simulink model "HexrotorDynamicModel_2015a"  (Simulink 8.5)
settings: Solver=ode45  SolverMode=SingleTasking  StartTime=0.0  StopTime=10  FixedStep=0.0001  RelTol=1e-3
values from neighbouring files (symbols this model uses):
  alpha = pi/180 * 13.6    (= 0.237364778271)    [IdealParameter.m]    (also in ParLuk11.m = deg2rad(13.6); Parameter.m = [-alpha_i;alpha_i;-alpha_i;alpha_i;-alpha_i;alpha_i]; ParameterIdeal.m = [-alpha_i;alpha_i;-alpha_i;alpha_i;-alpha_i;alpha_i]; ParameterVIVE.m = [alpha_i;-alpha_i;alpha_i;-alpha_i;alpha_i;-alpha_i])
  b = 1.1e-06    [IdealParameter.m]    (also in ParLuk11.m = 1.14e-07; Parameter.m = 8.944e-07; ParameterIdeal.m; ParameterVIVE.m)
  beta = 0    [IdealParameter.m]    (also in ParLuk11.m; Parameter.m = [beta_i; beta_i; beta_i; beta_i; beta_i; beta_i]; ParameterIdeal.m = [beta_i; beta_i; beta_i; beta_i; beta_i; beta_i]; ParameterVIVE.m = [beta_i; beta_i; beta_i; beta_i; beta_i; beta_i])
  g = 9.81    [IdealParameter.m]    (also in ParLuk11.m; Parameter.m; ParameterIdeal.m; ParameterVIVE.m)
  IB = [Ixx 0 0; 0 Iyy 0; 0 0 Izz]    [IdealParameter.m]    (also in ParLuk11.m; Parameter.m; ParameterIdeal.m; ParameterVIVE.m)
  k = 5.6e-05    [IdealParameter.m]    (also in ParLuk11.m = 2.98e-06; Parameter.m = 4.472e-05; ParameterIdeal.m; ParameterVIVE.m = 5.13e-05)
  k_ad = 4    [ParLuk11.m]
  k_ap = 2    [ParLuk11.m]
  K_d = diag([5,5,5,6,6,6])    [ParLuk11.m]
  K_p1 = 10*eye(3)    [ParLuk11.m]
  k_p2 = 6    [ParLuk11.m]
  K_P_1 = 15*eye(3)    [IdealParameter.m]    (also in ParLuk11.m = 6*eye(3); Parameter.m = 2*eye(3); ParameterIdeal.m; ParameterVIVE.m = 10*eye(3))
  K_P_2 = 50*eye(3)    [IdealParameter.m]    (also in ParLuk11.m = 6*eye(3); Parameter.m = 4*eye(3); ParameterIdeal.m; ParameterVIVE.m = 10*eye(3))
  K_P_3 = 60*eye(3)    [IdealParameter.m]    (also in ParLuk11.m = 6*eye(3); Parameter.m = 6*eye(3); ParameterIdeal.m; ParameterVIVE.m = 10*eye(3))
  K_P_D = 30*eye(3)    [IdealParameter.m]    (also in ParLuk11.m = 10*eye(3); Parameter.m = 5*eye(3); ParameterIdeal.m; ParameterVIVE.m = 15*eye(3))
  K_P_I = 100*eye(3)    [IdealParameter.m]    (also in ParLuk11.m = 10*eye(3); Parameter.m = 10*eye(3); ParameterIdeal.m = 80*eye(3); ParameterVIVE.m)
  K_P_P = 100*eye(3)    [IdealParameter.m]    (also in ParLuk11.m = 10*eye(3); Parameter.m = 10*eye(3); ParameterIdeal.m = 130*eye(3); ParameterVIVE.m)
  k_pd = 8    [ParLuk11.m]
  k_pp = 4    [ParLuk11.m]
  K_R_1 = 40*eye(3)    [IdealParameter.m]    (also in ParLuk11.m = 3*eye(3); Parameter.m = 2*eye(3); ParameterIdeal.m; ParameterVIVE.m = 10*eye(3))
  K_R_2 = 100*eye(3)    [IdealParameter.m]    (also in ParLuk11.m = 3*eye(3); Parameter.m = 4*eye(3); ParameterIdeal.m; ParameterVIVE.m = 10*eye(3))
  K_R_3 = 50*eye(4)    [IdealParameter.m]    (also in ParLuk11.m = eye(4); Parameter.m = 6*eye(4); ParameterIdeal.m; ParameterVIVE.m = 10*eye(4))
  K_R_D = 30*eye(3)    [IdealParameter.m]    (also in ParLuk11.m = 10*eye(3); Parameter.m = 5*eye(3); ParameterIdeal.m; ParameterVIVE.m = 15*eye(3))
  K_R_I = 100*eye(3)    [IdealParameter.m]    (also in ParLuk11.m = 10*eye(3); Parameter.m = 10*eye(3); ParameterIdeal.m = 80*eye(3); ParameterVIVE.m)
  K_R_P = 100*eye(3)    [IdealParameter.m]    (also in ParLuk11.m = 20*eye(3); Parameter.m = 10*eye(3); ParameterIdeal.m = 130*eye(3); ParameterVIVE.m)
  k_z = 15    [ParLuk11.m]
  L = 0.4    [IdealParameter.m]    (also in ParLuk11.m = 1; Parameter.m; ParameterIdeal.m; ParameterVIVE.m = 0.6)
  m = 1    [Controllability.m]    (also in IdealParameter.m = 2.5; ParLuk11.m = 0.6; Parameter.m = 4.85; ParameterIdeal.m = 4.85)
libraries: vrlib x8, simulink x3, dspmtrx3 x2
(part 2 of 2)

== matlab function Motion Equations/MATLAB Function1 ==
  data: w input double; Q output double
function Q = omegaSkew(w)
%#codegen

Q = [0 w(3) -w(2) w(1);
    -w(3) 0 w(1) w(2);
    w(2) -w(1) 0 w(3);
    -w(1) -w(2) -w(3) 0];

== matlab function Motion Equations/MATLAB Function2 ==
  data: R input double; RT output double
function RT = transpose(R)
%#codegen

RT = R';

== matlab function Feedback Linearization Control [Raj15]/MATLAB Function1 ==
  data: R_m input double; JR output double; I_B input double
function JR = computeJR(R_m, I_B)
JR = [R_m zeros(3);
     zeros(3) inv(I_B) ];

== matlab function Geometric Control on SE(3) [Ras17]/MATLAB Function ==
  data: W_g input double; W_ff output double; I input double; T_B input double; T_D input double; T_D_dot input double; H_er input double
function W_ff = computeW_ff(W_g, I, T_B, T_D, T_D_dot, H_er)

R_er = H_er(1:3,1:3);
eta_er = H_er(1:3,4);

%H_er_inv = [R_er', -R_er'*eta_er; 0,0,0,1];

Ad_H_er_inv = [R_er', zeros(3);
               vec2skew(-R_er'*eta_er)*R_er', R_er'];

T_er = T_B - Ad_H_er_inv*T_D;

ad_T_er = [vec2skew(T_er(1:3)), zeros(3);
            vec2skew(T_er(4:6)), vec2skew(T_er(1:3))];
        
ad_T_B = [vec2skew(T_B(1:3)), zeros(3);
    vec2skew(T_B(4:6)), vec2skew(T_B(1:3))];
        
W_ff =  - W_g ...
        - ad_T_B' * (I*T_B) ...
        + I * ( Ad_H_er_inv * T_D_dot - ad_T_er * Ad_H_er_inv * T_D);

== matlab function Geometric Control on SE(3) [Ras17]/MATLAB Function1 ==
  data: R_BtoI input double; g input double; W_g output double; m input double
function W_g = computeW_g(R_BtoI, g, m)

W_g = [R_BtoI', zeros(3);
        zeros(3), R_BtoI'] * [0,0,0,0,0,-m*g]';

== matlab function MATLAB Function2 ==
  data: t input double; p_d output double; p_d_dot output double; p_d_dotdot output double; R_d output double; omega_d output double; omega_d_dot output double; T_D output double; T_D_dot output double
function [p_d, p_d_dot, p_d_dotdot, R_d, omega_d, omega_d_dot, T_D, T_D_dot] = createTrajectory(t)

xa = 0;
xe = 5;
te = 5;
x = xa + 10*(xe-xa)*t^3/te^3 - 15*(xe-xa)*t^4/te^4 + 6*(xe-xa)*t^5/te^5;
x_dot = 3*10*(xe-xa)*t^2/te^3 - 4*15*(xe-xa)*t^3/te^4 + 5*6*(xe-xa)*t^4/te^5;
x_dot_dot = 6*10*(xe-xa)*t/te^3 - 12*15*(xe-xa)*t^2/te^4 + 20*6*(xe-xa)*t^3/te^5;
if (t> te)
    x = xe;
    x_dot = 0;
    x_dot_dot = 0;
end
p_d = [x;0;x];
p_d_dot = [x_dot;0;x_dot];
p_d_dotdot = [x_dot_dot;0;x_dot_dot];

ct = cos(2*pi/te*t);
st = sin(2*pi/te*t);
R_d = [ct, -st, 0; 
       st, ct, 0;
       0 0 1];
R_d_dot = [-st, -ct, 0;
            ct, -st, 0;
            0 0 0];
R_d_dotdot = [-ct, st, 0;
               -st, -ct, 0;
               0 0 0];
           
T_d_tilde = [R_d', -R_d'*p_d; 0,0,0,1]*[R_d_dot p_d_dot; 0,0,0,0];

omega_d = skew2vec(T_d_tilde(1:3,1:3));

T_d_tilde_dot = [R_d_dot'*R_d_dot+R_d'*R_d_dotdot, R_d_dot'*p_d_dot+R_d'*p_d_dotdot;
    0,0,0,0];

omega_d_dot = skew2vec(T_d_tilde_dot(1:3,1:3));

T_D = [omega_d; T_d_tilde(1:3,4)];
T_D_dot = [omega_d_dot; T_d_tilde_dot(1:3,4)];

if t>te
    R_d = eye(3);
    omega_d = [0;0;0];
    omega_d_dot = [0;0;0];
    T_D = zeros(6,1);
    T_D_dot = zeros(6,1);
end

%zeros
% 
% p_d = [0;0;0];
% p_d_dot = [0;0;0];
% p_d_dotdot = [0;0;0];
% R_d = eye(3);
% omega_d = [0;0;0];
% omega_d_dot = [0;0;0];
% T_D = zeros(6,1);
% T_D_dot = zeros(6,1);

== matlab function Geometric Control on SE(3) [Ras17]/MATLAB Function2 ==
  data: m input double; IB input double; I output double
function I = computeI(m, IB)

I = [IB, zeros(3); 
    zeros(3), eye(3)*m];

== matlab function Geometric Control on SE(3) [Ras17]/MATLAB Function3 ==
  data: R_BtoI input double; v_I input double; T_B output double; omega_B input double
function T_B = computeTB(R_BtoI, v_I, omega_B)

T_B = [omega_B;
    R_BtoI' * v_I];

== matlab function DC Motor Dynamics /MATLAB Function ==
  data: u input double; y output double
function y = fcn(u)

y = sqrt(abs(u))*sign(u);

== matlab function DC Motor Dynamics /MATLAB Function1 ==
  data: u input double; y output double
function y = fcn(u)

y = u^2*sign(u);

== matlab function DC Motor Dynamics /MATLAB Function2 ==
  data: u input double; y output double
function y = fcn(u)

y = sqrt(abs(u))*sign(u);

== matlab function DC Motor Dynamics /MATLAB Function3 ==
  data: u input double; y output double
function y = fcn(u)

y = u^2*sign(u);

== matlab function Feedback Linearization Control [Raj15]/MATLAB Function3 ==
  data: u input double; y output double
function y = transpose(u)

y = u';

== matlab function Feedback Linearization Control [Raj15]/MATLAB Function5 ==
  data: R_d input double; e_R output double; R_BtoI input double
function e_R = compute_e_R(R_d, R_BtoI)

A = R_d' * R_BtoI - R_BtoI' * R_d;

e_R = 0.5 * [A(3,2); A(1,3); A(2,1)];

== matlab function Geometric Control on SE(3) [Ras17]/MATLAB Function4 ==
  data: R_BtoI input double; H_er output double; R_d input double; p_I input double; p_d input double
function H_er = computeH_er(R_BtoI, R_d, p_I, p_d)

H_er = [R_d'*R_BtoI, R_d'*(p_I-p_d); 0,0,0,1];

== matlab function Geometric Control on SE(3) [Ras17]/MATLAB Function5 ==
  data: H_er input double; K_p1 input double; W_p output double; kp2 input double
function W_p = computeW_p(H_er, K_p1, kp2)

R_er = H_er(1:3,1:3);
eta_er = H_er(1:3,4);

W_p = - [skew2vec(0.5*(K_p1*R_er-(K_p1*R_er)'));
        -kp2*R_er'*eta_er];

== matlab function Geometric Control on SE(3) [Ras17]/MATLAB Function6 ==
  data: T_B input double; T_er output double; H_er input double; T_D input double
function T_er = computeT_er(T_B, H_er, T_D)

R_er = H_er(1:3,1:3);
eta_er = H_er(1:3,4);

Ad_H_er_inv = [R_er', zeros(3);
               vec2skew(-R_er'*eta_er)*R_er', R_er'];
           
T_er = T_B - Ad_H_er_inv * T_D;

== matlab function Geometric Control on SE(3) [Ras17]/MATLAB Function7 ==
  data: T_er input double; W_d output double; K_d input double
function W_d = compute_Wd(T_er,K_d)

W_d = - K_d * T_er;

== matlab function Geometric Control on SE(3) [Ras17]/MATLAB Function8 ==
  data: W input double; FH input double; u output double
function u = mapToRotors(W,FH)

u = inv(FH)*W;

== matlab function Motion Equations [Ras17]/MATLAB Function1 ==
  data: R_BtoI input double; g input double; W_g output double; m input double
function W_g = computeW_g(R_BtoI, g, m)

W_g = [R_BtoI', zeros(3);
        zeros(3), R_BtoI'] * [0,0,0,0,0,-m*g]';

== matlab function Motion Equations [Ras17]/MATLAB Function2 ==
  data: m input double; IB input double; I output double
function I = computeI(m, IB)

I = [IB, zeros(3); 
    zeros(3), eye(3)*m];

== matlab function Motion Equations [Ras17]/MATLAB Function ==
  data: I input double; Iinv output double
function Iinv = computeInverse(I)
Iinv = inv(I);

== matlab function Motion Equations [Ras17]/MATLAB Function3 ==
  data: T_B input double; ad_T_B output double
function ad_T_B = compute_ad_T_B(T_B)
ad_T_B = [vec2skew(T_B(1:3)), zeros(3);
    vec2skew(T_B(4:6)), vec2skew(T_B(1:3))]';

== matlab function Motion Equations [Ras17]/MATLAB Function4 ==
  data: R input double; RT output double
function RT = transpose(R)
%#codegen

RT = R';

== matlab function Motion Equations [Ras17]/MATLAB Function5 ==
  data: T input double; T_tilde output double
function T_tilde = computeT_tilde(T)

T_tilde = [vec2skew(T(1:3)), T(4:6); 0,0,0,0];

== matlab function Motion Equations [Ras17]/MATLAB Function6 ==
  data: H input double; R_BtoI output double; eta_BtoI output double
function [R_BtoI, eta_BtoI] = computeRandeta(H)

R_BtoI = H(1:3,1:3);
eta_BtoI = H(1:3,4);

== matlab function Zero Moment Control [Mic17] unfertig/MATLAB Function ==
  data: F1 input double; d output double; b2 output double; F2 input double; F2K output double
function [d,b2, F2K] = fcn(F1,F2)
    % null space of F2 or H: 
    % w01 = [1 0 0 1 0 0]', w02 = [0 1 0 0 1 0]', w03 = [0 0 1 0 0 1]'
    b2 = [1 1 1 1 1 1]'*1/2.4495;
    d = F1*b2;

    %null space of F1
    K1 = [-1 0 0; 0 -1 0; 0 0 -1; 1 0 0; 0 1 0; 0 0 1];
    
    % K = K1*K1'
    
    K = K1*K1';
    
    %K*F2'*inv(F2*K*F2');
    F2K = K*F2'/(F2*K*F2');

== matlab function Zero Moment Control [Mic17] unfertig/MATLAB Function1 ==
  data: w_d input double; Q output double
function Q = omegaSkew(w_d)
%#codegen

Q = [0 w_d(3) -w_d(2) w_d(1);
    -w_d(3) 0 w_d(1) w_d(2);
    w_d(2) -w_d(1) 0 w_d(3);
    -w_d(1) -w_d(2) -w_d(3) 0];

== matlab function Zero Moment Control [Mic17] unfertig/MATLAB Function2 ==
  data: q input double; R output double
function R = Quat2R(q)
% compute R from quaternion input

R = [q(1)^2 - q(2)^2 - q(3)^2 + q(4)^2,  2*(q(1)*q(2) - q(3)*q(4)),          2*(q(1)*q(3) + q(2)*q(4));
     2*(q(1)*q(2) + q(3)*q(4)),         -q(1)^2 + q(2)^2 - q(3)^2 + q(4)^2,  2*(q(2)*q(3) - q(1)*q(4));
     2*(q(1)*q(3) - q(2)*q(4)),          2*(q(2)*q(3) + q(1)*q(4)),         -q(1)^2 - q(2)^2 + q(3)^2 + q(4)^2];

== matlab function Zero Moment Control [Mic17] unfertig/MATLAB Function3 ==
  data: R input double; RT output double
function RT = transpose(R)
%#codegen

RT = R';

== matlab function Zero Moment Control [Mic17] unfertig/MATLAB Function4 ==
  data: f_p input double; w_d output double; Rqd input double; u_z input double
function w_d = compute_w_d(f_p, Rqd, u_z)

if f_p == 0
    f_p = 0.0001;
end
w_d = 1/f_p * vec2skew(Rqd) * u_z;

== matlab function Zero Moment Control [Mic17] unfertig/MATLAB Function5 ==
  data: k_pd input double; u_z output double; k_pp input double; k_z input double; m input double; e_p input double; e_v input double; z input double; d input double
function u_z = compute_u_z(k_pd, k_pp, k_z, m, e_p, e_v, z, d)

u_z = (k_pd*k_pp/m*e_p + (k_pd^2/m - k_pp)*e_v + (k_pd/m - k_z)*z)/norm(d, 2)^2;

== matlab function Zero Moment Control [Mic17] unfertig/MATLAB Function6 ==
  data: q input double; delta_q output double; q_d input double
function delta_q = compute_deltaq(q, q_d)

eps_d = q_d(1:3);
n_d = q_d(4);
eps_q = q(1:3);
n_q = q(4);

delta_n = n_d*n_q + eps_d'*eps_q;
delta_eps = -n_q*eps_d + n_d*eps_q - vec2skew(eps_d)*eps_q;

delta_q = [delta_eps; delta_n];

== matlab function Zero Moment Control [Mic17] unfertig/MATLAB Function7 ==
  data: f_p input double; w_dd output double; R_qd input double; d input double; k_pd input double; k_pp input double; m input double; R_q input double; e_p input double; e_v input double; kz input double; z input double
function w_dd = compute_wdd(f_p,R_qd,d, k_pd, k_pp, m, R_q, e_p, e_v, kz,z)

x = (k_pd^2/m^2 - k_pp/m)*(R_q*d*f_p-k_pp*e_p) + ...
    (2*k_pp*k_pd/m - k_pd^3/m^2)*e_v + (k_pd^2/m^2 - k_pp/m - k_pd*kz/m + kz^2)*z;

w_dd = 1/f_p *1/(norm(d)^2) * vec2skew(R_qd*d) * x;

== matlab function Zero Moment Control [Mic17] unfertig/MATLAB Function8 ==
  data: k_ap input double; tau_r output double; k_ad input double; q_delta input double; Rq input double; w_d input double; w input double; J input double; w_dd input double
function tau_r = compute_tau_r(k_ap, k_ad, q_delta, Rq, w_d, w, J, w_dd)

delta_eps = q_delta(1:3);

tau_r = -k_ap*delta_eps - k_ad * (w - Rq'*w_d) + cross(w, J*w) ...
    - J*vec2skew(w)*Rq'*w_d + J*Rq'*w_dd;

== matlab function Integral Backstepping/MATLAB Function1 ==
  data: R input double; q output double
function q   = DCM2Quat(R)

%%%%%%%%%%%%%%%%%%%%%%%%%%%%%%%%%%%%%%%%%%%%%%%%%%%%%%%%%%%%%%%%%%%%%%%%%%%
%
% M-file: Tool_DCM2Quat
%         -> impelmeted as M-Function
% Author: Marcel Tkocz
% Version: 27.01.2008
%
% Description:
%   This Function converts roll-pitch-yaw angels into their quaternion
%   equivalents.
%
% Inputs:
%   Orientation ... orientation in roll-pitch-yaw angels
%
% Outputs:
%   q           ... orientation in quaternions
%   
%%%%%%%%%%%%%%%%%%%%%%%%%%%%%%%%%%%%%%%%%%%%%%%%%%%%%%%%%%%%%%%%%%%%%%%%%%%

%--------------------------------------------------------------------------
% Calculation of Quaternions based on q1
%--------------------------------------------------------------------------
q = [0 0 0 1]';

if (1 + R(1,1) - R(2,2) - R(3,3)) > 0 
    q1 = 1/2*sqrt(1 + R(1,1) - R(2,2) - R(3,3));
    q2 = 1/(4*q1)*( R(1,2) + R(2,1));
    q3 = 1/(4*q1)*( R(1,3) + R(3,1));
    q4 = 1/(4*q1)*(-R(2,3) + R(3,2));

    if round(q1) ~= 0
        q = [q1; q2; q3; q4];
    end
end

%--------------------------------------------------------------------------
% Calculation of Quaternions based on q2
%--------------------------------------------------------------------------

if (1 - R(1,1) + R(2,2) - R(3,3)) > 0
    q2 = 1/2*sqrt(1 - R(1,1) + R(2,2) - R(3,3));
    q1 = 1/(4*q2)*( R(1,2) + R(2,1));
    q3 = 1/(4*q2)*( R(2,3) + R(3,2));
    q4 = 1/(4*q2)*( R(1,3) - R(3,1));

    if round(q2) ~= 0
        q = [q1; q2; q3; q4];
    end
end

%--------------------------------------------------------------------------
% Calculation of Quaternions based on q3
%--------------------------------------------------------------------------

if (1 - R(1,1) - R(2,2) + R(3,3)) > 0
    q3 = 1/2*sqrt(1 - R(1,1) - R(2,2) + R(3,3));
    q1 = 1/(4*q3)*( R(1,3) + R(3,1));
    q2 = 1/(4*q3)*( R(2,3) + R(3,2));
    q4 = 1/(4*q3)*(-R(1,2) + R(2,1));

    if round(q3) ~= 0
        q = [q1; q2; q3; q4];
    end
end

%--------------------------------------------------------------------------
% Calculation of Quaternions based on q4
%--------------------------------------------------------------------------

if (1 + R(1,1) + R(2,2) + R(3,3)) > 0
    q4 = 1/2*sqrt(1 + R(1,1) + R(2,2) + R(3,3));
    q1 = 1/(4*q4)*(-R(2,3) + R(3,2));
    q2 = 1/(4*q4)*(-R(3,1) + R(1,3));
    q3 = 1/(4*q4)*(-R(1,2) + R(2,1));

    if round(q4) ~= 0
        q = [q1; q2; q3; q4];
    end
end


end

== matlab function Integral Backstepping/MATLAB Function ==
  data: epsilon_d input double; eta_d input double; epsilon input double; eta input double; eta_tilde output double; epsilon_tilde output double; epsilon_tilde_T output double; skew_eps_tilde output double
function [eta_tilde, epsilon_tilde, epsilon_tilde_T, skew_eps_tilde] = calc_q_tilde(epsilon_d, eta_d, epsilon, eta)

eta_tilde = eta_d*eta + epsilon_d'*epsilon;

epsilon_tilde = eta * epsilon_d - eta_d*epsilon - vec2skew(epsilon_d)*epsilon;

epsilon_tilde_T = epsilon_tilde';

skew_eps_tilde = vec2skew(epsilon_tilde);

== matlab function Integral Backstepping/MATLAB Function2 ==
  data: eta_tilde input double; z1 output double; eps_tilde input double
function z1 = compute_z1(eta_tilde, eps_tilde)

z1 = [1-abs(eta_tilde);
    eps_tilde];

== matlab function Integral Backstepping/MATLAB Function3 ==
  data: eta_tilde input double; G output double; eps_tilde input double
function G = compute_G(eta_tilde, eps_tilde)

if (eta_tilde >= 0)
    sig = 1;
else
    sig = -1;
end

G = [sig*eps_tilde';
    eye(3)*eta_tilde + vec2skew(eps_tilde)]';

== matlab function Integral Backstepping/MATLAB Function4 ==
  data: K1 input double; alpha_dot output double; G input double; z1 input double; z2 input double; omega_tilde input double; eta_tilde input double; eps_tilde input double; K3 input double; Xsi input double
function alpha_dot = compute_alpha_dot(K1,G,z1,z2, omega_tilde, eta_tilde, eps_tilde, K3, Xsi)

eta_dot = -0.5*eps_tilde'*omega_tilde;

eps_dot = 0.5*(eta_tilde*eye(3) + vec2skew(eps_tilde))*omega_tilde;

if eta_tilde >= 0
    sig = 1;
else
    sig = -1;
end

G_dot = [sig*eps_dot';
        eta_dot*eye(3) + vec2skew(eps_dot)]';

% alpha_dot = -K1 ( G_dot * z1 + G * z1_dot) 
% - 2 (-inv(GT)G_dot inv(GT) * K3 * Xsi + inv(GT)K3*z1
alpha_dot1 = -K1*(G_dot*z1  + G*(-0.5*G'*K1*G*z1 + 0.5*G'*z2));

pGT = pinv(G.');

alpha_dot2 = -2*(-pGT*(G_dot.')*pGT*K3*Xsi + pGT*K3*z1);

alpha_dot=alpha_dot1+ alpha_dot2;

== matlab function Integral Backstepping/MATLAB Function5 ==
  data: J input double; J_inv output double
function J_inv = inverse(J)

J_inv = inv(J);

== matlab function Integral Backstepping/MATLAB Function6 ==
  data: R_m input double; JR output double; I_B input double
function JR = computeJR(R_m, I_B)
JR = [R_m zeros(3);
     zeros(3) inv(I_B) ];

== matlab function Integral Backstepping/MATLAB Function7 ==
  data: R input double; q output double
function q   = DCM2Quat(R)

%%%%%%%%%%%%%%%%%%%%%%%%%%%%%%%%%%%%%%%%%%%%%%%%%%%%%%%%%%%%%%%%%%%%%%%%%%%
%
% M-file: Tool_DCM2Quat
%         -> impelmeted as M-Function
% Author: Marcel Tkocz
% Version: 27.01.2008
%
% Description:
%   This Function converts roll-pitch-yaw angels into their quaternion
%   equivalents.
%
% Inputs:
%   Orientation ... orientation in roll-pitch-yaw angels
%
% Outputs:
%   q           ... orientation in quaternions
%   
%%%%%%%%%%%%%%%%%%%%%%%%%%%%%%%%%%%%%%%%%%%%%%%%%%%%%%%%%%%%%%%%%%%%%%%%%%%

%--------------------------------------------------------------------------
% Calculation of Quaternions based on q1
%--------------------------------------------------------------------------
q = [0 0 0 1]';

if (1 + R(1,1) - R(2,2) - R(3,3)) > 0 
    q1 = 1/2*sqrt(1 + R(1,1) - R(2,2) - R(3,3));
    q2 = 1/(4*q1)*( R(1,2) + R(2,1));
    q3 = 1/(4*q1)*( R(1,3) + R(3,1));
    q4 = 1/(4*q1)*(-R(2,3) + R(3,2));

    if round(q1) ~= 0
        q = [q1; q2; q3; q4];
    end
end

%--------------------------------------------------------------------------
% Calculation of Quaternions based on q2
%--------------------------------------------------------------------------

if (1 - R(1,1) + R(2,2) - R(3,3)) > 0
    q2 = 1/2*sqrt(1 - R(1,1) + R(2,2) - R(3,3));
    q1 = 1/(4*q2)*( R(1,2) + R(2,1));
    q3 = 1/(4*q2)*( R(2,3) + R(3,2));
    q4 = 1/(4*q2)*( R(1,3) - R(3,1));

    if round(q2) ~= 0
        q = [q1; q2; q3; q4];
    end
end

%--------------------------------------------------------------------------
% Calculation of Quaternions based on q3
%--------------------------------------------------------------------------

if (1 - R(1,1) - R(2,2) + R(3,3)) > 0
    q3 = 1/2*sqrt(1 - R(1,1) - R(2,2) + R(3,3));
    q1 = 1/(4*q3)*( R(1,3) + R(3,1));
    q2 = 1/(4*q3)*( R(2,3) + R(3,2));
    q4 = 1/(4*q3)*(-R(1,2) + R(2,1));

    if round(q3) ~= 0
        q = [q1; q2; q3; q4];
    end
end

%--------------------------------------------------------------------------
% Calculation of Quaternions based on q4
%--------------------------------------------------------------------------

if (1 + R(1,1) + R(2,2) + R(3,3)) > 0
    q4 = 1/2*sqrt(1 + R(1,1) + R(2,2) + R(3,3));
    q1 = 1/(4*q4)*(-R(2,3) + R(3,2));
    q2 = 1/(4*q4)*(-R(3,1) + R(1,3));
    q3 = 1/(4*q4)*(-R(1,2) + R(2,1));

    if round(q4) ~= 0
        q = [q1; q2; q3; q4];
    end
end


end

== matlab function Feedback Linearization Control [Raj15]/MATLAB Function2 ==
  data: I input double; I_inv output double
function I_inv = inverse(I)

I_inv = inv(I);

== matlab function Motion Equations/MATLAB Function3 ==
  data: I input double; I_inv output double
function I_inv = inverse(I)

I_inv = inv(I);

== matlab function Motion Equations, p_I/MATLAB Function3 ==
  data: I input double; I_inv output double
function I_inv = inverse(I)

I_inv = inv(I);

== matlab function Integral Backstepping/MATLAB Function8 ==
  data: I input double; I_inv output double
function I_inv = inverse(I)

I_inv = inv(I);

== matlab function Backstepping1/MATLAB Function ==
  data: epsilon_d input double; eta_d input double; epsilon input double; eta input double; eta_tilde output double; epsilon_tilde output double; epsilon_tilde_T output double; skew_eps_tilde output double
function [eta_tilde, epsilon_tilde, epsilon_tilde_T, skew_eps_tilde] = calc_q_tilde(epsilon_d, eta_d, epsilon, eta)

eta_tilde = eta_d*eta + epsilon_d'*epsilon;

epsilon_tilde = eta * epsilon_d - eta_d*epsilon - vec2skew(epsilon_d)*epsilon;

epsilon_tilde_T = epsilon_tilde';

skew_eps_tilde = vec2skew(epsilon_tilde);

== matlab function Backstepping1/MATLAB Function1 ==
  data: R input double; q output double
function q   = DCM2Quat(R)

%%%%%%%%%%%%%%%%%%%%%%%%%%%%%%%%%%%%%%%%%%%%%%%%%%%%%%%%%%%%%%%%%%%%%%%%%%%
%
% M-file: Tool_DCM2Quat
%         -> impelmeted as M-Function
% Author: Marcel Tkocz
% Version: 27.01.2008
%
% Description:
%   This Function converts roll-pitch-yaw angels into their quaternion
%   equivalents.
%
% Inputs:
%   Orientation ... orientation in roll-pitch-yaw angels
%
% Outputs:
%   q           ... orientation in quaternions
%   
%%%%%%%%%%%%%%%%%%%%%%%%%%%%%%%%%%%%%%%%%%%%%%%%%%%%%%%%%%%%%%%%%%%%%%%%%%%

%--------------------------------------------------------------------------
% Calculation of Quaternions based on q1
%--------------------------------------------------------------------------
q = [0 0 0 1]';

if (1 + R(1,1) - R(2,2) - R(3,3)) > 0 
    q1 = 1/2*sqrt(1 + R(1,1) - R(2,2) - R(3,3));
    q2 = 1/(4*q1)*( R(1,2) + R(2,1));
    q3 = 1/(4*q1)*( R(1,3) + R(3,1));
    q4 = 1/(4*q1)*(-R(2,3) + R(3,2));

    if round(q1) ~= 0
        q = [q1; q2; q3; q4];
    end
end

%--------------------------------------------------------------------------
% Calculation of Quaternions based on q2
%--------------------------------------------------------------------------

if (1 - R(1,1) + R(2,2) - R(3,3)) > 0
    q2 = 1/2*sqrt(1 - R(1,1) + R(2,2) - R(3,3));
    q1 = 1/(4*q2)*( R(1,2) + R(2,1));
    q3 = 1/(4*q2)*( R(2,3) + R(3,2));
    q4 = 1/(4*q2)*( R(1,3) - R(3,1));

    if round(q2) ~= 0
        q = [q1; q2; q3; q4];
    end
end

%--------------------------------------------------------------------------
% Calculation of Quaternions based on q3
%--------------------------------------------------------------------------

if (1 - R(1,1) - R(2,2) + R(3,3)) > 0
    q3 = 1/2*sqrt(1 - R(1,1) - R(2,2) + R(3,3));
    q1 = 1/(4*q3)*( R(1,3) + R(3,1));
    q2 = 1/(4*q3)*( R(2,3) + R(3,2));
    q4 = 1/(4*q3)*(-R(1,2) + R(2,1));

    if round(q3) ~= 0
        q = [q1; q2; q3; q4];
    end
end

%--------------------------------------------------------------------------
% Calculation of Quaternions based on q4
%--------------------------------------------------------------------------

if (1 + R(1,1) + R(2,2) + R(3,3)) > 0
    q4 = 1/2*sqrt(1 + R(1,1) + R(2,2) + R(3,3));
    q1 = 1/(4*q4)*(-R(2,3) + R(3,2));
    q2 = 1/(4*q4)*(-R(3,1) + R(1,3));
    q3 = 1/(4*q4)*(-R(1,2) + R(2,1));

    if round(q4) ~= 0
        q = [q1; q2; q3; q4];
    end
end


end

== matlab function Backstepping1/MATLAB Function2 ==
  data: eta_tilde input double; z1 output double; eps_tilde input double
function z1 = compute_z1(eta_tilde, eps_tilde)

z1 = [1-abs(eta_tilde);
    eps_tilde];

== matlab function Backstepping1/MATLAB Function3 ==
  data: eta_tilde input double; G output double; eps_tilde input double
function G = compute_G(eta_tilde, eps_tilde)

if (eta_tilde >= 0)
    sig = 1;
else
    sig = -1;
end

G = [sig*eps_tilde';
    eye(3)*eta_tilde + vec2skew(eps_tilde)]';

== matlab function Backstepping1/MATLAB Function4 ==
  data: K1 input double; alpha_dot output double; G input double; z1 input double; z2 input double; omega_tilde input double; eta_tilde input double; eps_tilde input double
function alpha_dot = compute_alpha_dot(K1,G,z1,z2, omega_tilde, eta_tilde, eps_tilde)

eta_dot = -0.5*eps_tilde'*omega_tilde;

eps_dot = 0.5*(eta_tilde*eye(3) + vec2skew(eps_tilde))*omega_tilde;

if eta_tilde >= 0
    sig = 1;
else
    sig = -1;
end

G_dot = [sig*eps_dot';
        eta_dot*eye(3) + vec2skew(eps_dot)]';

% alpha_dot = -K1 ( G_dot * z1 + G * z1_dot)
alpha_dot = -K1*(G_dot*z1  + G*(-0.5*G'*K1*G*z1 + 0.5*G'*z2));

== matlab function Backstepping1/MATLAB Function5 ==
  data: J input double; J_inv output double
function J_inv = inverse(J)

J_inv = inv(J);

== matlab function Backstepping1/MATLAB Function6 ==
  data: R_m input double; JR output double; I_B input double
function JR = computeJR(R_m, I_B)
JR = [R_m zeros(3);
     zeros(3) inv(I_B) ];

== matlab function Backstepping1/MATLAB Function7 ==
  data: R input double; q output double
function q   = DCM2Quat(R)

%%%%%%%%%%%%%%%%%%%%%%%%%%%%%%%%%%%%%%%%%%%%%%%%%%%%%%%%%%%%%%%%%%%%%%%%%%%
%
% M-file: Tool_DCM2Quat
%         -> impelmeted as M-Function
% Author: Marcel Tkocz
% Version: 27.01.2008
%
% Description:
%   This Function converts roll-pitch-yaw angels into their quaternion
%   equivalents.
%
% Inputs:
%   Orientation ... orientation in roll-pitch-yaw angels
%
% Outputs:
%   q           ... orientation in quaternions
%   
%%%%%%%%%%%%%%%%%%%%%%%%%%%%%%%%%%%%%%%%%%%%%%%%%%%%%%%%%%%%%%%%%%%%%%%%%%%

%--------------------------------------------------------------------------
% Calculation of Quaternions based on q1
%--------------------------------------------------------------------------
q = [0 0 0 1]';

if (1 + R(1,1) - R(2,2) - R(3,3)) > 0 
    q1 = 1/2*sqrt(1 + R(1,1) - R(2,2) - R(3,3));
    q2 = 1/(4*q1)*( R(1,2) + R(2,1));
    q3 = 1/(4*q1)*( R(1,3) + R(3,1));
    q4 = 1/(4*q1)*(-R(2,3) + R(3,2));

    if round(q1) ~= 0
        q = [q1; q2; q3; q4];
    end
end

%--------------------------------------------------------------------------
% Calculation of Quaternions based on q2
%--------------------------------------------------------------------------

if (1 - R(1,1) + R(2,2) - R(3,3)) > 0
    q2 = 1/2*sqrt(1 - R(1,1) + R(2,2) - R(3,3));
    q1 = 1/(4*q2)*( R(1,2) + R(2,1));
    q3 = 1/(4*q2)*( R(2,3) + R(3,2));
    q4 = 1/(4*q2)*( R(1,3) - R(3,1));

    if round(q2) ~= 0
        q = [q1; q2; q3; q4];
    end
end

%--------------------------------------------------------------------------
% Calculation of Quaternions based on q3
%--------------------------------------------------------------------------

if (1 - R(1,1) - R(2,2) + R(3,3)) > 0
    q3 = 1/2*sqrt(1 - R(1,1) - R(2,2) + R(3,3));
    q1 = 1/(4*q3)*( R(1,3) + R(3,1));
    q2 = 1/(4*q3)*( R(2,3) + R(3,2));
    q4 = 1/(4*q3)*(-R(1,2) + R(2,1));

    if round(q3) ~= 0
        q = [q1; q2; q3; q4];
    end
end

%--------------------------------------------------------------------------
% Calculation of Quaternions based on q4
%--------------------------------------------------------------------------

if (1 + R(1,1) + R(2,2) + R(3,3)) > 0
    q4 = 1/2*sqrt(1 + R(1,1) + R(2,2) + R(3,3));
    q1 = 1/(4*q4)*(-R(2,3) + R(3,2));
    q2 = 1/(4*q4)*(-R(3,1) + R(1,3));
    q3 = 1/(4*q4)*(-R(1,2) + R(2,1));

    if round(q4) ~= 0
        q = [q1; q2; q3; q4];
    end
end


end

== matlab function Backstepping1/MATLAB Function8 ==
  data: I input double; I_inv output double
function I_inv = inverse(I)

I_inv = inv(I);

== matlab function Integral Backstepping/MATLAB Function9 ==
  data: K1 input double; alpha output double; G input double; z1 input double; K3 input double; Xsi input double
function alpha = compute_alpha(K1,G,z1,K3,Xsi)

alpha = -K1*G*z1 - 2*pinv(G.')*K3*Xsi;

== matlab function Zero Moment Control [Mic17] unfertig/MATLAB Function9 ==
  data: R input double; q output double
function q   = DCM2Quat(R)

%%%%%%%%%%%%%%%%%%%%%%%%%%%%%%%%%%%%%%%%%%%%%%%%%%%%%%%%%%%%%%%%%%%%%%%%%%%
%
% M-file: Tool_DCM2Quat
%         -> impelmeted as M-Function
% Author: Marcel Tkocz
% Version: 27.01.2008
%
% Description:
%   This Function converts roll-pitch-yaw angels into their quaternion
%   equivalents.
%
% Inputs:
%   Orientation ... orientation in roll-pitch-yaw angels
%
% Outputs:
%   q           ... orientation in quaternions
%   
%%%%%%%%%%%%%%%%%%%%%%%%%%%%%%%%%%%%%%%%%%%%%%%%%%%%%%%%%%%%%%%%%%%%%%%%%%%

%--------------------------------------------------------------------------
% Calculation of Quaternions based on q1
%--------------------------------------------------------------------------
q = [0 0 0 1]';

if (1 + R(1,1) - R(2,2) - R(3,3)) > 0 
    q1 = 1/2*sqrt(1 + R(1,1) - R(2,2) - R(3,3));
    q2 = 1/(4*q1)*( R(1,2) + R(2,1));
    q3 = 1/(4*q1)*( R(1,3) + R(3,1));
    q4 = 1/(4*q1)*(-R(2,3) + R(3,2));

    if round(q1) ~= 0
        q = [q1; q2; q3; q4];
    end
end

%--------------------------------------------------------------------------
% Calculation of Quaternions based on q2
%--------------------------------------------------------------------------

if (1 - R(1,1) + R(2,2) - R(3,3)) > 0
    q2 = 1/2*sqrt(1 - R(1,1) + R(2,2) - R(3,3));
    q1 = 1/(4*q2)*( R(1,2) + R(2,1));
    q3 = 1/(4*q2)*( R(2,3) + R(3,2));
    q4 = 1/(4*q2)*( R(1,3) - R(3,1));

    if round(q2) ~= 0
        q = [q1; q2; q3; q4];
    end
end

%--------------------------------------------------------------------------
% Calculation of Quaternions based on q3
%--------------------------------------------------------------------------

if (1 - R(1,1) - R(2,2) + R(3,3)) > 0
    q3 = 1/2*sqrt(1 - R(1,1) - R(2,2) + R(3,3));
    q1 = 1/(4*q3)*( R(1,3) + R(3,1));
    q2 = 1/(4*q3)*( R(2,3) + R(3,2));
    q4 = 1/(4*q3)*(-R(1,2) + R(2,1));

    if round(q3) ~= 0
        q = [q1; q2; q3; q4];
    end
end

%--------------------------------------------------------------------------
% Calculation of Quaternions based on q4
%--------------------------------------------------------------------------

if (1 + R(1,1) + R(2,2) + R(3,3)) > 0
    q4 = 1/2*sqrt(1 + R(1,1) + R(2,2) + R(3,3));
    q1 = 1/(4*q4)*(-R(2,3) + R(3,2));
    q2 = 1/(4*q4)*(-R(3,1) + R(1,3));
    q3 = 1/(4*q4)*(-R(1,2) + R(2,1));

    if round(q4) ~= 0
        q = [q1; q2; q3; q4];
    end
end


end
